simulink subsystem "SD_2nd_Order_Modulator"  (R2022b)
settings: Solver=VariableStepAuto  StartTime=0.0  StopTime=10.0  RelTol=1e-3
settings Model: Creator=1111293  LastModifiedBy=qaztr
settings SolverCC: AlgebraicLoopSolver=TrustRegion
settings DebuggingCC: UnconnectedInputMsg=warning  UnconnectedOutputMsg=warning  UnconnectedLineMsg=warning  SFMachineParentedDataDiag=warning
settings ModelReferenceCC: EnableRefExpFcnMdlSchedulingChecks=on
settings RTWCC: DLArmComputeVersion=19.05

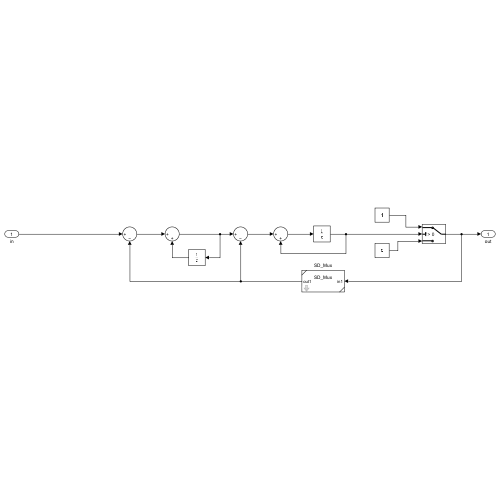
[thumbnail: Simulink's stored preview of the top-level diagram]
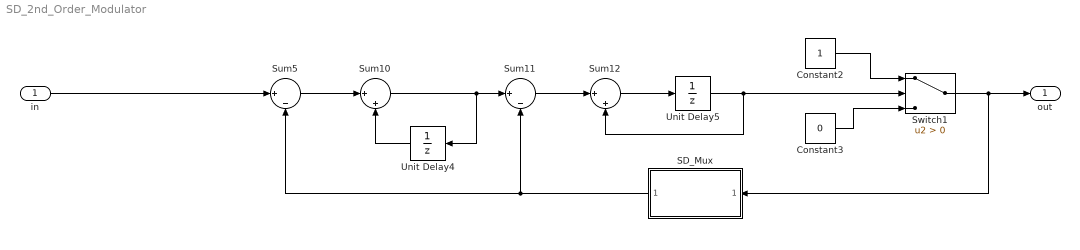
== system SD_2nd_Order_Modulator ==
  in : Inport
  Constant2 : Constant  OutDataTypeStr=boolean
  Constant3 : Constant  Value=0  OutDataTypeStr=boolean
  SD_Mux : Subsystem  ReferencedSubsystem=SD_Mux  a=sd_mod_amp  Parameter2=fixdt(1,32,23)
  Sum10 : Sum  Inputs=||+|+  OutDataTypeStr=Inherit: Same as accumulator
  Sum11 : Sum  Inputs=||+|-  OutDataTypeStr=Inherit: Same as accumulator
  Sum12 : Sum  Inputs=||+|+  OutDataTypeStr=Inherit: Same as accumulator
  Sum5 : Sum  Inputs=||+|-  OutDataTypeStr=Inherit: Same as accumulator
  Switch1 : Switch  Criteria=u2 > Threshold  SaturateOnIntegerOverflow=off  InputSameDT=off
  Unit Delay4 : UnitDelay  SampleTime=-1  HasFrameUpgradeWarning=on
  Unit Delay5 : UnitDelay  SampleTime=-1  HasFrameUpgradeWarning=on
  out : Outport
  wires:
  Sum5/1 -> Sum10/1
  Unit Delay4/1 -> Sum10/2
  Sum10/1 -> Sum11/1, Unit Delay4/1
  Sum11/1 -> Sum12/1
  Unit Delay5/1 -> Sum12/2, Switch1/2
  Sum12/1 -> Unit Delay5/1
  in/1 -> Sum5/1
  Constant3/1 -> Switch1/3
  Constant2/1 -> Switch1/1
  SD_Mux/1 -> Sum5/2, Sum11/2
  Switch1/1 -> out/1, SD_Mux/1
